simulink model "Turbine"  (R2024b)
settings: Solver=VariableStepAuto  StartTime=0.0  StopTime=100  RelTol=1e-3
undefined symbols (not defined in the file): DiscIntNeverNeededParam
libraries: nesl_utility x6, fl_lib x5, simulink x1, ee_lib x1
settings Model: Creator=Msi  LastModifiedBy=Msi

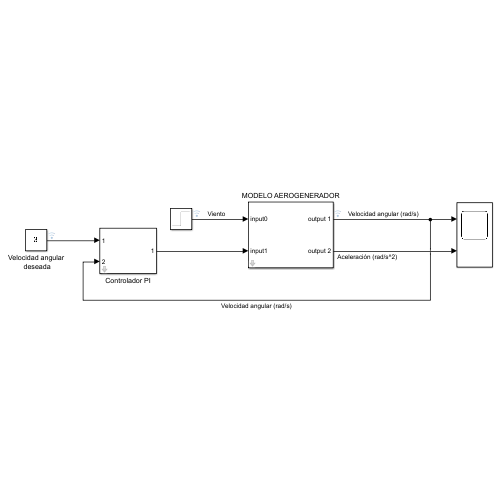
[thumbnail: Simulink's stored preview of the top-level diagram]
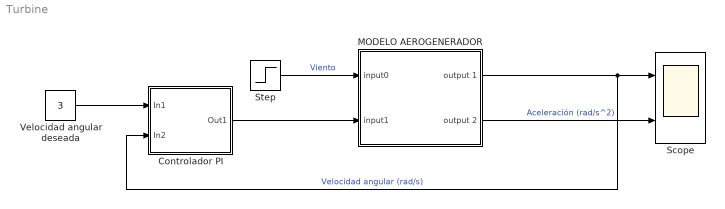
== system Turbine ==
  Controlador PI : Subsystem  mask{Kp=2.8, Ki=1}
      mask prompts: Kp "Ganancia Proporcional"; Ki "Ganancia Integral"
  MODELO AEROGENERADOR : Subsystem  mask{Torque_Generador=-1e6, Inercia=1.6e8}
      mask prompts: Torque_Generador "Torque de freno debido al generador (Debe ser un valor negativo en Nm)"; Inercia "Inercia del rotor de la turbina (kg*m^2)"
  Scope : Scope  NumInputPorts=2
  Step : Step  Time=60  Before=30  After=30  SampleTime=0
  Velocidad angular deseada : Constant  Value=3
  wires:
  Step/1 -> MODELO AEROGENERADOR/1(input0)  "Viento"
  MODELO AEROGENERADOR/1(output 1) -> Scope/1, Controlador PI/2(In2)  "Velocidad angular (rad/s)"
  MODELO AEROGENERADOR/2(output 2) -> Scope/2  "Aceleración (rad/s^2)"
  Velocidad angular deseada/1 -> Controlador PI/1(In1)
  Controlador PI/1(Out1) -> MODELO AEROGENERADOR/2(input1)

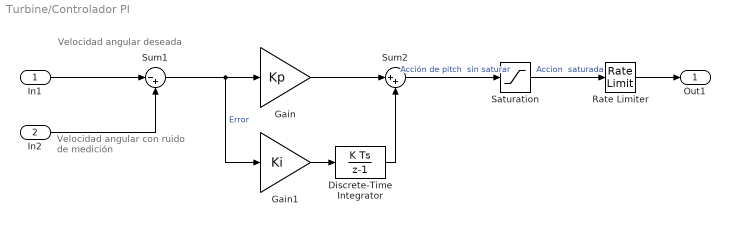
== system Turbine/Controlador PI ==
  note: Velocidad angular
      | con ruido de medición
  note: Velocidad angular
      | deseada
  In1 : Inport
  In2 : Inport  Port=2
  Discrete-Time Integrator : DiscreteIntegrator  SampleTime=0.01  LimitOutput=on  UpperSaturationLimit=90  LowerSaturationLimit=0  ICPrevOutput=DiscIntNeverNeededParam  ICPrevScaledInput=DiscIntNeverNeededParam
  Gain : Gain  Gain=Kp
  Gain1 : Gain  Gain=Ki
  Rate Limiter : RateLimiter  RisingSlewLimit=10  FallingSlewLimit=-10  SampleTimeMode=inherited
  Saturation : Saturate  UpperLimit=90  LowerLimit=0
  Sum1 : Sum  Inputs=|-+
  Sum2 : Sum  Inputs=|++
  Out1 : Outport
  wires:
  In1/1 -> Sum1/1
  In2/1 -> Sum1/2
  Sum1/1 -> Gain1/1, Gain/1  "Error"
  Gain1/1 -> Discrete-Time Integrator/1
  Saturation/1 -> Rate Limiter/1  "Accion  saturada"
  Discrete-Time Integrator/1 -> Sum2/2
  Sum2/1 -> Saturation/1  "Acción de pitch  sin saturar"
  Gain/1 -> Sum2/1
  Rate Limiter/1 -> Out1/1

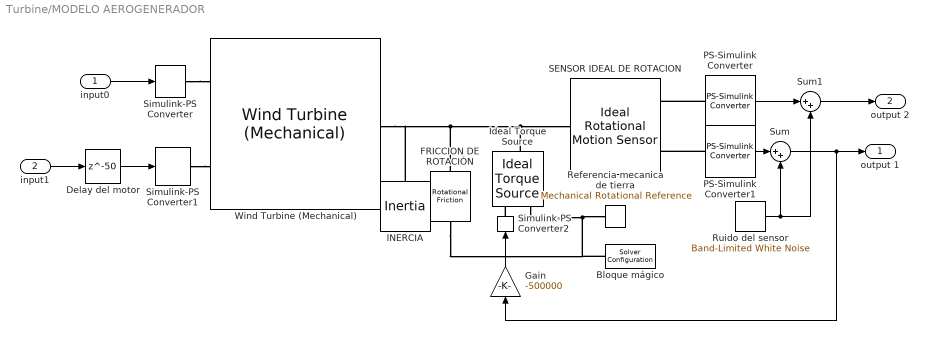
== system Turbine/MODELO AEROGENERADOR ==
  input0 : Inport
  input1 : Inport  Port=2
  Bloque mágico : nesl_utility/Solver Configuration  PhysicalDomain=network_engine_domain  SubClassName=solver  LeftPortType=input  RightPortType=generic  Tones=[]  Harmonics=[]  SimulateNoise=off  Profile=off  UseLocalSampling=off  EnableSwitchedLinearOptims=on  FrequencyDomain=off  UseCCode=off  RelTol=0.001  AbsTol=0.001  MinStep=1e-09  ToWorkspace=off  RevertToSquareIcSolve=off  NumHomotopyIterations=100  PhasorMode=off  PhasorModeNumHarmonics=1  ConsistencySolver=NEWTON_XTOL_AFTER_FTOL  IndexReductionMethod=DerivativeReplacement  DoDC=off  ResidualTolerance=1e-09  ConsistencyTolSource=GLOBAL  ConsistencyAbsTol=0.001  ConsistencyRelTol=0.001  ConsistencyTolFactor=0.001  UseLocalSolver=off  LocalSolverChoice=NE_BACKWARD_EULER_ADVANCER  ResolveIndetEquations=on  FunctionEvalNumThread=1  LocalSolverSampleTime=0.001  DoFixedCost=off  MaxNonlinIter=3  MaxModeIter=2  ComputeImpulses=off  ImpulseIterations=2  LinearAlgebra=auto  LinearAlgebraNumThread=0  EquationFormulation=NE_TIME_EF  DelaysMemoryBudget=1024  AutomaticFiltering=on  FilteringTimeConstant=0.001  PartitionStorageMethod=AS_NEEDED  PartitionMemoryBudget=1024  PartitionMethod=ROBUST  MultibodyUseLocalSolver=off  MultibodyLocalSolverChoice=ODE1  MultibodyLocalSolverSampleTime=0.001
  Delay del motor : Delay  DelayLength=50  InitialCondition=0  SampleTime=0.01
  FRICCION DE ROTACIÓN : fl_lib/Mechanical/Rotational Elements/Rotational Friction  brkwy_trq=25 N*m  brkwy_vel=0.1 rad/s  Col_trq=20 N*m  visc_coef=0.001 N*m*s/rad  w_specify=off  w_priority=None  w=0 rad/s  w_nominal_specify=off  w_nominal_value=1  w_nominal_unit=rad/s  t_specify=off  t_priority=None  t=0 N*m  t_nominal_specify=off  t_nominal_value=1  t_nominal_unit=N*m
  Gain : Gain  Gain=-500000
  INERCIA : fl_lib/Mechanical/Rotational Elements/Inertia  inertia=Inercia kg*m^2  num_ports=foundation.enum.numPorts2.one  w_specify=off  w_priority=High  w=0 rad/s  w_nominal_specify=off  w_nominal_value=1  w_nominal_unit=rad/s  t_specify=off  t_priority=None  t=0 N*m  t_nominal_specify=off  t_nominal_value=1  t_nominal_unit=N*m
  Ideal Torque Source : fl_lib/Mechanical/Mechanical Sources/Ideal Torque Source
  PS-Simulink Converter : nesl_utility/PS-Simulink Converter  PhysicalDomain=network_engine_domain  SubClassName=ps_output  LeftPortType=input  RightPortType=output  PseudoPeriodic=off  Frequencies=[]  VectorFormat=inherit  Unit=inherit  AffineConversion=off
  PS-Simulink Converter1 : nesl_utility/PS-Simulink Converter  PhysicalDomain=network_engine_domain  SubClassName=ps_output  LeftPortType=input  RightPortType=output  PseudoPeriodic=off  Frequencies=[]  VectorFormat=inherit  Unit=inherit  AffineConversion=off
  Referencia mecanica de tierra : fl_lib/Mechanical/Rotational Elements/Mechanical Rotational Reference
  Ruido del sensor : simulink/Sources/Band-Limited White Noise  Cov=[0.0000005]  Ts=0.01  seed=[23341]
  SENSOR IDEAL DE ROTACION : fl_lib/Mechanical/Mechanical Sensors/Ideal Rotational Motion Sensor  reference=foundation.enum.MeasurementReference.absolute  acceleration_port=true  velocity_port=true  position_port=false  wrap_angle=false  offset=0 rad
      settings: InternalSimscapePortConfiguration="{\"Bottom\":[],\"Left\":[{\"id\":\"R\",\"label\":\"R\",\"type\":\"foundation.mechanical.rotational.rotational\"}],\"Right\":[{\"id\":\"alpha\",\"label\":\"α\",\"type\":\"output\"},{\"id\":\"W\",\"label\":\"W\",\"type\":\"output\"}],\"Top\":[]}"
  Simulink-PS Converter : nesl_utility/Simulink-PS Converter  PhysicalDomain=network_engine_domain  SubClassName=ps_input  LeftPortType=input  RightPortType=output  PseudoPeriodic=off  Frequencies=[]  NoiseDistribution=none  NoiseParameters=[]  Unit=1  AffineConversion=off  FilteringAndDerivatives=provide  SimscapeFilterOrder=1  InputFilterTimeConstant=0.001  UdotUserProvided=0
  Simulink-PS Converter1 : nesl_utility/Simulink-PS Converter  PhysicalDomain=network_engine_domain  SubClassName=ps_input  LeftPortType=input  RightPortType=output  PseudoPeriodic=off  Frequencies=[]  NoiseDistribution=none  NoiseParameters=[]  Unit=1  AffineConversion=off  FilteringAndDerivatives=provide  SimscapeFilterOrder=1  InputFilterTimeConstant=0.001  UdotUserProvided=0
  Simulink-PS Converter2 : nesl_utility/Simulink-PS Converter  PhysicalDomain=network_engine_domain  SubClassName=ps_input  LeftPortType=input  RightPortType=output  PseudoPeriodic=off  Frequencies=[]  NoiseDistribution=none  NoiseParameters=[]  Unit=1  AffineConversion=off  FilteringAndDerivatives=provide  SimscapeFilterOrder=1  InputFilterTimeConstant=0.001  UdotUserProvided=0
  Sum : Sum  Inputs=|++
  Sum1 : Sum  Inputs=|++
  Wind Turbine (Mechanical) : ee_lib/Electromechanical/Wind Turbine (Mechanical)  R_rotor=80 m  pitch_TLU=[0, 3, 5, 10, 20, 90] deg  lambda_TLU=[0, 2, 4, 6, 8, 10, 12, 14, 15]  Cp_TLU=[0.0010, 0.0161, 0.1446, 0.3865, 0.5009, 0.4404, 0.2545, 0.0002, -0.1384; 0.0016, 0.0173, 0.1079, 0.2676, 0.3779, 0.4111, 0.3838, 0.3176, 0.2753; 0.0027, 0.0197, 0.1151, 0.2606, 0.3469, 0.3558, 0.3069, 0.2222, 0.1718; 0.0054, 0.0283, 0.1315, 0.2364, 0.2589, 0.2022, 0.0929, -0.0455, -0.1204; 0.0109, 0.0536, 0.1320, 0.1256, 0.0120, -0.1752, -0.4017, -0.6435, -0.7655; -0.01 * ones(1, 9)]  v_thr=0.01 m/s  w_thr=0.01 rad/s  rho_air=1.225 kg/m^3  includeInertia=false  J=5e6 kg*m^2  lam=0 N*m*s/rad  w_specify=off  w_priority=None  w=0 rad/s  w_nominal_specify=off  w_nominal_value=1  w_nominal_unit=rad/s  t_specify=off  t_priority=None  t=0 N*m  t_nominal_specify=off  t_nominal_value=1  t_nominal_unit=N*m  Torque_specify=off  Torque_priority=None  Torque=0 N*m  Torque_nominal_specify=off  Torque_nominal_value=1  Torque_nominal_unit=N*m
      settings: InternalSimscapePortConfiguration="{\"Bottom\":[],\"Left\":[{\"id\":\"vWind\",\"label\":\"V\",\"type\":\"input\"},{\"id\":\"pitch\",\"label\":\"β\",\"type\":\"input\"}],\"Right\":[{\"id\":\"R\",\"label\":\"R\",\"type\":\"foundation.mechanical.rotational.rotational\"}],\"Top\":[]}"
  output 1 : Outport
  output 2 : Outport  Port=2
  wires:
  input0/1 -> Simulink-PS Converter/1
  Gain/1 -> Simulink-PS Converter2/1
  input1/1 -> Delay del motor/1
  Delay del motor/1 -> Simulink-PS Converter1/1
  Sum1/1 -> output 2/1
  PS-Simulink Converter1/1 -> Sum/1
  Ruido del sensor/1 -> Sum/2, Sum1/2
  Sum/1 -> Gain/1, output 1/1
  PS-Simulink Converter/1 -> Sum1/1
  connections:
  Ideal Torque Source/RConn2 -- Bloque mágico/RConn1 -- FRICCION DE ROTACIÓN/RConn1 -- Referencia mecanica de tierra/LConn1
  PS-Simulink Converter/LConn1 -- SENSOR IDEAL DE ROTACION/RConn1
  Ideal Torque Source/LConn1 -- INERCIA/LConn1 -- Wind Turbine (Mechanical)/RConn1 -- FRICCION DE ROTACIÓN/LConn1 -- SENSOR IDEAL DE ROTACION/LConn1
  Simulink-PS Converter2/RConn1 -- Ideal Torque Source/RConn1
  Simulink-PS Converter/RConn1 -- Wind Turbine (Mechanical)/LConn1
  Simulink-PS Converter1/RConn1 -- Wind Turbine (Mechanical)/LConn2
  PS-Simulink Converter1/LConn1 -- SENSOR IDEAL DE ROTACION/RConn2
